simulink model "SimulationModel_VR_Sink"  (R2014a)
settings: Solver=ode3  SolverMode=SingleTasking  StartTime=0.0  StopTime=180  FixedStep=deltaT  RelTol=1e-3
PostLoadFcn:
  | loadRobotParameters
  | 
  | allotedRunTime = 3*60; % [sec] Time allowed for run
  | 
  | % starting parameters
  | % The timer starts once the robot has moved a certain distance from the
  | % starting point
  | startPos = [50 50]; % [cm]
  | startingRadius = 10; % [cm]
  | 
  | % Target parameters
  | targetBoundaryRadius = 7; % [cm] radius considered at location
  | statTimeReq = 2.5; % [sec] minimum time robot must be at location
InitFcn:
  | close('all','force');
StartFcn:
  | reset(SimDisplay.getInstance());
undefined symbols (not defined in the file or in its folder): AxleLength, deltaT, dT, EncL_init, EncR_init, EncRes, gray, motorBiasLeft, motorBiasRight, motorDeadZoneFwd, motorDeadZoneRev, motorGainLeft, motorGainRight, Rec, SDTV, TargetPositions, theta0, Ts, WheelRadius, x0, y0
libraries: vrlib x7, simulink x5, visionsinks x2, opclib x1, visiontextngfix x1, visionconversions x1, visionanalysis x1, simulink_extras x1, aerolibtransform2 x1
(part 2 of 2)

== matlab function SimulationModel_VR_Sink/RobotModel/relative_to_targets ==
  data: robotPos input size=[1 2]; hCam input; alphaCam input; robotTheta input size=1; dist output; bearing output; targetsPos input; pcam output; lcam output
function [dist,bearing, pcam ,lcam] = targets(robotPos,hCam,alphaCam,robotTheta,targetsPos)
%#codegen
%% TARGETS Returns distance and bearing for each target relative to robot
%
% Distances and positions are in cm
% Angles are in degrees
%
% Inputs
%   - hCam: Cam height (from ground)
%   - targetsPos: Position of targets (X,Y)
%   - robotPos: Robot position (X,Y)
%   - robotTheta: Robot angle
%
% Outputs
%   - dist (array nx1 with n=nb targets): Distances for each target, 
%       if a target cannot be seen by the camera associated distance 
%       is equal to -1
%   - bearing (array nx1 with n=nb targets): Angles for each target, 
%       if a target cannot be seen by the camera associated angle is 
%       equal to -1
%

% Get camera field of vision
% [pcam,lcam]=camera(hCam);
% betaCam = 21 ;
% etaCam = 27 ;
% [pcam, lcam] = cameraAnalytic(hCam,90-alphaCam, betaCam, etaCam);
pcam = [25, 105];
lcam = [27, 108];

% Convert target position to robot reference
[x,y] = world2robot(robotPos(1),robotPos(2),robotTheta,targetsPos(:,1),targetsPos(:,2));

% Get distance and bearing for each point relative to robot
[dist,bearing] = isincamera(pcam,lcam,x,y);


function [p_cam,l_cam]=camera(h_camera)
%% CAMERA Returns camera field of vision
%
% Input
%   - h_camera: Camera height (in cm)
%
% Outputs
%   - p_cam: Camera vision depth, 2 values: minimal and maximal depth for 
%       the camera position. Depth corresponds to Y axis. Unit = cm.
%   - l_cam: Camera vision width, 2 values: minimal and maximal width for 
%       the camera position. Width corresponds to X axis. Unit = cm.
%

% Calibration values
% ------------------
% Height
height=[10 23 41 52];
% Depth
pmin=[13 34 40 50];
pmax=[100 160 240 300];
% Width
lmin=[20 50 62 62];
lmax=[110 205 300 360];

% Polynomial approximation with 1rst degree polynom (y = a*x+b)
coef_pmin=polyfit(height(2:end),pmin(2:end),1);
coef_pmax=polyfit(height(2:end),pmax(2:end),1);
coef_lmin=polyfit(height(2:end),lmin(2:end),1);
coef_lmax=polyfit(height(2:end),lmax(2:end),1);

% Depth and width are calculated with polynomial approximation
p_cam=[ polyval(coef_pmin,h_camera) polyval(coef_pmax,h_camera)];
l_cam=[ polyval(coef_lmin,h_camera) polyval(coef_lmax,h_camera)];


function [p_cam, l_cam] = cameraAnalytic(h_camera, alpha_camera, beta_camera, eta_camera)
%
%
% Inputs
%   - h_camera      : Camera height (in cm)
%   - alpha_camera  : angle between the vertical (z-axis) and the camera 
%   - beta_camera   : vertical angle of view of camera / 2 (in degrees)
%   - eta_camera    : horizontal angle of view of camera / 2 (in degrees)
%
% Outputs
%   - p_cam: Camera vision depth, 2 values: minimal and maximal depth for 
%       the camera position. Depth corresponds to Y axis. Unit = cm.
%   - l_cam: Camera vision width, 2 values: minimal and maximal width for 
%       the camera position. Width corresponds to X axis. Unit = cm.
%

l_cam = zeros(1,2);
p_cam = zeros(1,2);
d1 = h_camera * tand( alpha_camera + beta_camera ) ;
d2 = h_camera * tand( alpha_camera - beta_camera ) ;
k1 = h_camera / cosd( alpha_camera - beta_camera ) ;
k2 = h_camera / cosd( alpha_camera + beta_camera ) ;
f1 = k1 * tand( eta_camera ) ;
f2 = k2 * tand( eta_camera ) ;

l_cam(1) = 2 * f1 ;
l_cam(2) = 2 * f2 ;
p_cam(1) = d2 ;
p_cam(2) = d1 ;
p_far_factor = -7;
p_close_factor = 2;
p_cam(2) = p_cam(2) + p_far_factor;
p_cam(1) = p_cam(1) + p_close_factor;



function [x_new,y_new]=world2robot(x_robot,y_robot,theta_robot,x_world,y_world)
% WORLD2ROBOT Convert coordinates from world to robot
%
% Inputs
%   - x_robot: Robot X position (in world reference)
%   - y_robot: Robot Y position (in world reference)
%   - theta_robot: Robot angle  (in world reference)
%   - x_world: X value(s) to convert (in world reference)
%   - y_world: Y value(s) to convert (in world reference)
%
% Outpus
%   - x_new: Point(s) coordinate (X) in robot reference
%   - y_new: Point(s) coordinate (Y) in robot reference

% Translate coordinates reference
x_dif=x_world-x_robot;
y_dif=y_world-y_robot;

% Rotate coordinates reference
% x_new=x_dif*cosd(theta_robot)-y_dif*sind(theta_robot);
% y_new=x_dif*sind(theta_robot)+y_dif*cosd(theta_robot);
x_new = cosd(theta_robot)*x_dif + sind(theta_robot)*y_dif;
y_new = cosd(theta_robot)*y_dif - sind(theta_robot)*x_dif;
% see http://www.mathematics-online.org/inhalt/aussage/aussage444/

% TODO We have identified that the sign of converted coordinates is the
% opposite of the expected but we don't have an explanation for that
% x_new = -x_new;
% y_new = -y_new;

function [dist,bearing]=isincamera(p,l,x,y)
%% ISINCAMERA Distance and angle from current robot position
%
% Inputs
%   - p (2 elements vector): Minimal and maximal depth for camera (Y axis)
%   - l (2 elements vector): Minimal and maximal width for camera (X axis)
%   - x (vector): X coordinate of point(s)
%   - y (vector): Y coordinate of point(s)
%
% Outputs
%   - dist (vector): Distance of each point from camera (robot), -1 if
%       point cannot be seen by camera.
%   - bearing (vector): Angle of each point from camera (robot), -1 if
%       point cannot be seen by camera.
%

% Calculate coefficients for lines that defines the camera field of vision
% Field vision limits in Y axis are constants (y = p(1) or y = p(2))
c1=polyfit(p(1:2),[-l(1)/2 -l(2)/2],1);
c2=polyfit(p(1:2),[l(1)/2 l(2)/2],1);

% To be visible a point must match all the following criterion
%   - Y >= minimal depth
%   - Y <= maximal depth
%   - X >= - (width for current Y) / 2
%   - X <=   (width for current Y) / 2
%

%isvisible = y>=p(1) & y<=p(2) & (x>=polyval(c1,y) & x<=polyval(c2,y));
isvisible = x>=p(1) & x<=p(2) & (y>=polyval(c1,x) & y<=polyval(c2,x));

% Calculate distance and bearing for all points
dist = sqrt(x.^2 + y.^2);
% bearing = atan2d(y,x);
bearing = atan2d(x,-y)-90;

% Replace values by -1 for points that are not visible
dist(~isvisible) = 0;
bearing(~isvisible) = 0;

== matlab function SimulationModel_VR_Sink/RobotModel/dist_bearing2locatedTargets ==
  data: robotPos input; dist input; locatedTargets output; bearing input; robotTheta input
function locatedTargets = fcn(robotPos, dist, bearing, robotTheta)
%#codegen

loc = dist>0;

locatedTargetsX = zeros(size(dist));
locatedTargetsY = locatedTargetsX;

targetTheta = robotTheta+bearing(loc);

locatedTargetsX(loc) = robotPos(1)+dist(loc).*cosd(targetTheta);
locatedTargetsY(loc) = robotPos(2)+dist(loc).*sind(targetTheta);

locatedTargets = [locatedTargetsX, locatedTargetsY];

== matlab function SimulationModel_VR_Sink/RobotModel/CalculateRobotPosition/CalcPosFromWheelSpeeds ==
  data: wL input; wR input; x input; y input; theta input; dt input; xnew output; ynew output; thetanew output; AxleLength parameter; WheelRadius parameter
function [xnew,ynew, thetanew] = calcRobPos(wL, wR, x, y, theta, dt, AxleLength, WheelRadius)
%#codegen

vL = wL*WheelRadius;
vR = wR*WheelRadius;

if(vL == vR)
    xdot = vL * cos(theta);
    ydot = vR * sin(theta); 
    xnew = x + xdot*dt;
    ynew = y + ydot*dt;
    thetanew = theta;
else
    R = (AxleLength/2)*(vL + vR)/(vR - vL);
    omega = (vR - vL)/AxleLength;
    
    ICCx = x - R*sin(theta);
    ICCy = y + R*cos(theta);
    rotMat = [cos(omega*dt) -sin(omega*dt) 0;...
              sin(omega*dt) cos(omega*dt) 0;...
              0 0 1];
    newpos = rotMat*[x - ICCx; y-ICCy; theta] + [ICCx;ICCy;omega*dt];
    xnew = newpos(1);
    ynew = newpos(2);
    thetanew = newpos(3);
end

if thetanew > 2*pi
    thetanew = thetanew - (2*pi);
elseif thetanew < 0
    thetanew = thetanew + (2*pi);
end

end
